simulink model "control_pos_6dof_sinMI"  (R2023b)
settings: Solver=ode45  StartTime=0.0  StopTime=tsim  FixedStep=tstep  MaxStep=tstep  RelTol=tstep/10
undefined symbols (not defined in the file): a0, a1, robot_params, t_qeq_init, t_tr_init, tau_L, tr_ref
(part 2 of 7)

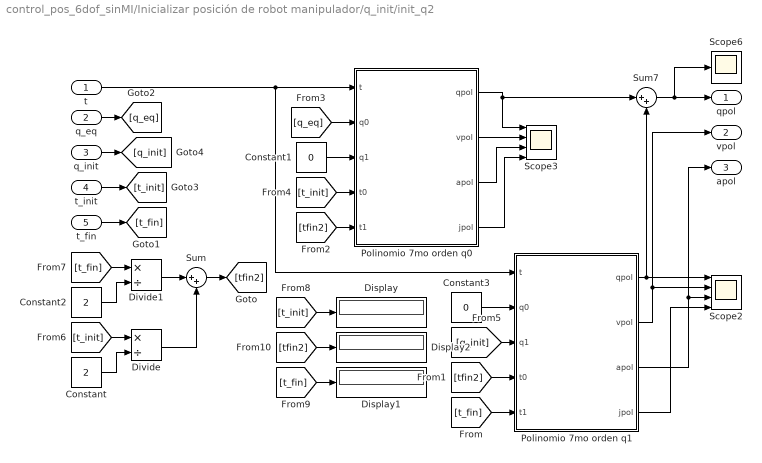
== system control_pos_6dof_sinMI/Inicializar posición de robot manipulador/q_init/init_q2 ==
  t : Inport
  q_eq : Inport  Port=2
  q_init : Inport  Port=3
  t_init : Inport  Port=4
  t_fin : Inport  Port=5
  Constant : Constant  Value=2
  Constant1 : Constant  Value=0
  Constant2 : Constant  Value=2
  Constant3 : Constant  Value=0
  Display : Display
  Display1 : Display
  Display2 : Display
  Divide : Product  Inputs=*/
  Divide1 : Product  Inputs=*/
  Polinomio 7mo orden q0 : MATLAB Function  TreatAsAtomicUnit=on
  Polinomio 7mo orden q1 : MATLAB Function  TreatAsAtomicUnit=on
  Scope2 : Scope  NumInputPorts=4
  Scope3 : Scope  NumInputPorts=4
  Scope6 : Scope
  Sum : Sum  Inputs=|++
  Sum7 : Sum  Inputs=|++
  qpol : Outport
  vpol : Outport  Port=2
  apol : Outport  Port=3
  wires:
  [tfin2] -> Polinomio 7mo orden q0/5(t1)
  t/1 -> Polinomio 7mo orden q1/1(t), Polinomio 7mo orden q0/1(t)
  t_fin/1 -> [t_fin]
  Polinomio 7mo orden q0/1(qpol) -> Sum7/1, Scope3/1
  Polinomio 7mo orden q1/1(qpol) -> Scope2/1, Sum7/2
  [tfin2] -> Polinomio 7mo orden q1/4(t0)
  [t_fin] -> Polinomio 7mo orden q1/5(t1)
  q_eq/1 -> [q_eq]
  q_init/1 -> [q_init]
  [q_eq] -> Polinomio 7mo orden q0/2(q0)
  [q_init] -> Polinomio 7mo orden q1/3(q1)
  Constant1/1 -> Polinomio 7mo orden q0/3(q1)
  Constant3/1 -> Polinomio 7mo orden q1/2(q0)
  Sum7/1 -> qpol/1, Scope6/1
  t_init/1 -> [t_init]
  [t_init] -> Polinomio 7mo orden q0/4(t0)
  Sum/1 -> [tfin2]
  [t_init] -> Display/1
  [t_fin] -> Display1/1
  [tfin2] -> Display2/1
  Divide/1 -> Sum/2
  Constant/1 -> Divide/2
  Divide1/1 -> Sum/1
  Constant2/1 -> Divide1/2
  [t_fin] -> Divide1/1
  [t_init] -> Divide/1
  Polinomio 7mo orden q1/2(vpol) -> vpol/1, Scope2/2
  Polinomio 7mo orden q1/3(apol) -> apol/1, Scope2/3
  Polinomio 7mo orden q1/4(jpol) -> Scope2/4
  Polinomio 7mo orden q0/2(vpol) -> Scope3/2
  Polinomio 7mo orden q0/3(apol) -> Scope3/3
  Polinomio 7mo orden q0/4(jpol) -> Scope3/4

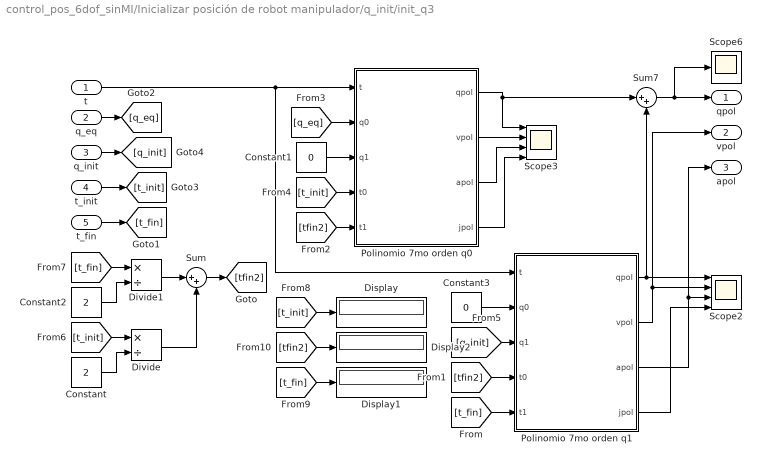
== system control_pos_6dof_sinMI/Inicializar posición de robot manipulador/q_init/init_q3 ==
  t : Inport
  q_eq : Inport  Port=2
  q_init : Inport  Port=3
  t_init : Inport  Port=4
  t_fin : Inport  Port=5
  Constant : Constant  Value=2
  Constant1 : Constant  Value=0
  Constant2 : Constant  Value=2
  Constant3 : Constant  Value=0
  Display : Display
  Display1 : Display
  Display2 : Display
  Divide : Product  Inputs=*/
  Divide1 : Product  Inputs=*/
  Polinomio 7mo orden q0 : MATLAB Function  TreatAsAtomicUnit=on
  Polinomio 7mo orden q1 : MATLAB Function  TreatAsAtomicUnit=on
  Scope2 : Scope  NumInputPorts=4
  Scope3 : Scope  NumInputPorts=4
  Scope6 : Scope
  Sum : Sum  Inputs=|++
  Sum7 : Sum  Inputs=|++
  qpol : Outport
  vpol : Outport  Port=2
  apol : Outport  Port=3
  wires:
  [tfin2] -> Polinomio 7mo orden q0/5(t1)
  t/1 -> Polinomio 7mo orden q1/1(t), Polinomio 7mo orden q0/1(t)
  t_fin/1 -> [t_fin]
  Polinomio 7mo orden q0/1(qpol) -> Sum7/1, Scope3/1
  Polinomio 7mo orden q1/1(qpol) -> Scope2/1, Sum7/2
  [tfin2] -> Polinomio 7mo orden q1/4(t0)
  [t_fin] -> Polinomio 7mo orden q1/5(t1)
  q_eq/1 -> [q_eq]
  q_init/1 -> [q_init]
  [q_eq] -> Polinomio 7mo orden q0/2(q0)
  [q_init] -> Polinomio 7mo orden q1/3(q1)
  Constant1/1 -> Polinomio 7mo orden q0/3(q1)
  Constant3/1 -> Polinomio 7mo orden q1/2(q0)
  Sum7/1 -> qpol/1, Scope6/1
  t_init/1 -> [t_init]
  [t_init] -> Polinomio 7mo orden q0/4(t0)
  Sum/1 -> [tfin2]
  [t_init] -> Display/1
  [t_fin] -> Display1/1
  [tfin2] -> Display2/1
  Divide/1 -> Sum/2
  Constant/1 -> Divide/2
  Divide1/1 -> Sum/1
  Constant2/1 -> Divide1/2
  [t_fin] -> Divide1/1
  [t_init] -> Divide/1
  Polinomio 7mo orden q1/2(vpol) -> vpol/1, Scope2/2
  Polinomio 7mo orden q1/3(apol) -> apol/1, Scope2/3
  Polinomio 7mo orden q1/4(jpol) -> Scope2/4
  Polinomio 7mo orden q0/2(vpol) -> Scope3/2
  Polinomio 7mo orden q0/3(apol) -> Scope3/3
  Polinomio 7mo orden q0/4(jpol) -> Scope3/4

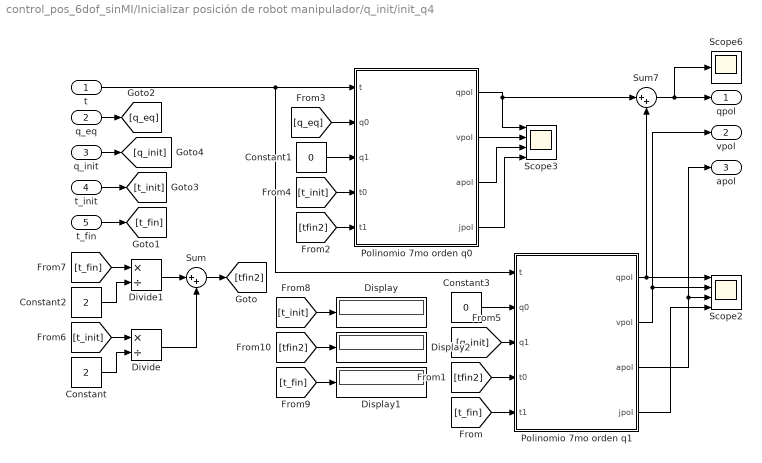
== system control_pos_6dof_sinMI/Inicializar posición de robot manipulador/q_init/init_q4 ==
  t : Inport
  q_eq : Inport  Port=2
  q_init : Inport  Port=3
  t_init : Inport  Port=4
  t_fin : Inport  Port=5
  Constant : Constant  Value=2
  Constant1 : Constant  Value=0
  Constant2 : Constant  Value=2
  Constant3 : Constant  Value=0
  Display : Display
  Display1 : Display
  Display2 : Display
  Divide : Product  Inputs=*/
  Divide1 : Product  Inputs=*/
  Polinomio 7mo orden q0 : MATLAB Function  TreatAsAtomicUnit=on
  Polinomio 7mo orden q1 : MATLAB Function  TreatAsAtomicUnit=on
  Scope2 : Scope  NumInputPorts=4
  Scope3 : Scope  NumInputPorts=4
  Scope6 : Scope
  Sum : Sum  Inputs=|++
  Sum7 : Sum  Inputs=|++
  qpol : Outport
  vpol : Outport  Port=2
  apol : Outport  Port=3
  wires:
  [tfin2] -> Polinomio 7mo orden q0/5(t1)
  t/1 -> Polinomio 7mo orden q1/1(t), Polinomio 7mo orden q0/1(t)
  t_fin/1 -> [t_fin]
  Polinomio 7mo orden q0/1(qpol) -> Sum7/1, Scope3/1
  Polinomio 7mo orden q1/1(qpol) -> Scope2/1, Sum7/2
  [tfin2] -> Polinomio 7mo orden q1/4(t0)
  [t_fin] -> Polinomio 7mo orden q1/5(t1)
  q_eq/1 -> [q_eq]
  q_init/1 -> [q_init]
  [q_eq] -> Polinomio 7mo orden q0/2(q0)
  [q_init] -> Polinomio 7mo orden q1/3(q1)
  Constant1/1 -> Polinomio 7mo orden q0/3(q1)
  Constant3/1 -> Polinomio 7mo orden q1/2(q0)
  Sum7/1 -> qpol/1, Scope6/1
  t_init/1 -> [t_init]
  [t_init] -> Polinomio 7mo orden q0/4(t0)
  Sum/1 -> [tfin2]
  [t_init] -> Display/1
  [t_fin] -> Display1/1
  [tfin2] -> Display2/1
  Divide/1 -> Sum/2
  Constant/1 -> Divide/2
  Divide1/1 -> Sum/1
  Constant2/1 -> Divide1/2
  [t_fin] -> Divide1/1
  [t_init] -> Divide/1
  Polinomio 7mo orden q1/2(vpol) -> vpol/1, Scope2/2
  Polinomio 7mo orden q1/3(apol) -> apol/1, Scope2/3
  Polinomio 7mo orden q1/4(jpol) -> Scope2/4
  Polinomio 7mo orden q0/2(vpol) -> Scope3/2
  Polinomio 7mo orden q0/3(apol) -> Scope3/3
  Polinomio 7mo orden q0/4(jpol) -> Scope3/4

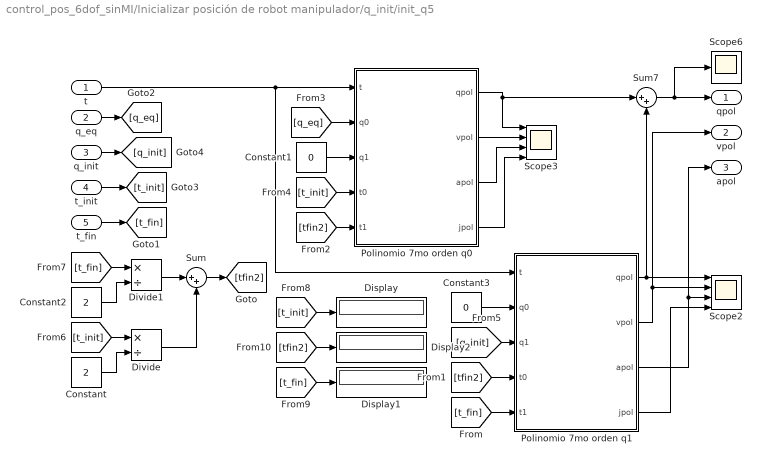
== system control_pos_6dof_sinMI/Inicializar posición de robot manipulador/q_init/init_q5 ==
  t : Inport
  q_eq : Inport  Port=2
  q_init : Inport  Port=3
  t_init : Inport  Port=4
  t_fin : Inport  Port=5
  Constant : Constant  Value=2
  Constant1 : Constant  Value=0
  Constant2 : Constant  Value=2
  Constant3 : Constant  Value=0
  Display : Display
  Display1 : Display
  Display2 : Display
  Divide : Product  Inputs=*/
  Divide1 : Product  Inputs=*/
  Polinomio 7mo orden q0 : MATLAB Function  TreatAsAtomicUnit=on
  Polinomio 7mo orden q1 : MATLAB Function  TreatAsAtomicUnit=on
  Scope2 : Scope  NumInputPorts=4
  Scope3 : Scope  NumInputPorts=4
  Scope6 : Scope
  Sum : Sum  Inputs=|++
  Sum7 : Sum  Inputs=|++
  qpol : Outport
  vpol : Outport  Port=2
  apol : Outport  Port=3
  wires:
  [tfin2] -> Polinomio 7mo orden q0/5(t1)
  t/1 -> Polinomio 7mo orden q1/1(t), Polinomio 7mo orden q0/1(t)
  t_fin/1 -> [t_fin]
  Polinomio 7mo orden q0/1(qpol) -> Sum7/1, Scope3/1
  Polinomio 7mo orden q1/1(qpol) -> Scope2/1, Sum7/2
  [tfin2] -> Polinomio 7mo orden q1/4(t0)
  [t_fin] -> Polinomio 7mo orden q1/5(t1)
  q_eq/1 -> [q_eq]
  q_init/1 -> [q_init]
  [q_eq] -> Polinomio 7mo orden q0/2(q0)
  [q_init] -> Polinomio 7mo orden q1/3(q1)
  Constant1/1 -> Polinomio 7mo orden q0/3(q1)
  Constant3/1 -> Polinomio 7mo orden q1/2(q0)
  Sum7/1 -> qpol/1, Scope6/1
  t_init/1 -> [t_init]
  [t_init] -> Polinomio 7mo orden q0/4(t0)
  Sum/1 -> [tfin2]
  [t_init] -> Display/1
  [t_fin] -> Display1/1
  [tfin2] -> Display2/1
  Divide/1 -> Sum/2
  Constant/1 -> Divide/2
  Divide1/1 -> Sum/1
  Constant2/1 -> Divide1/2
  [t_fin] -> Divide1/1
  [t_init] -> Divide/1
  Polinomio 7mo orden q1/2(vpol) -> vpol/1, Scope2/2
  Polinomio 7mo orden q1/3(apol) -> apol/1, Scope2/3
  Polinomio 7mo orden q1/4(jpol) -> Scope2/4
  Polinomio 7mo orden q0/2(vpol) -> Scope3/2
  Polinomio 7mo orden q0/3(apol) -> Scope3/3
  Polinomio 7mo orden q0/4(jpol) -> Scope3/4

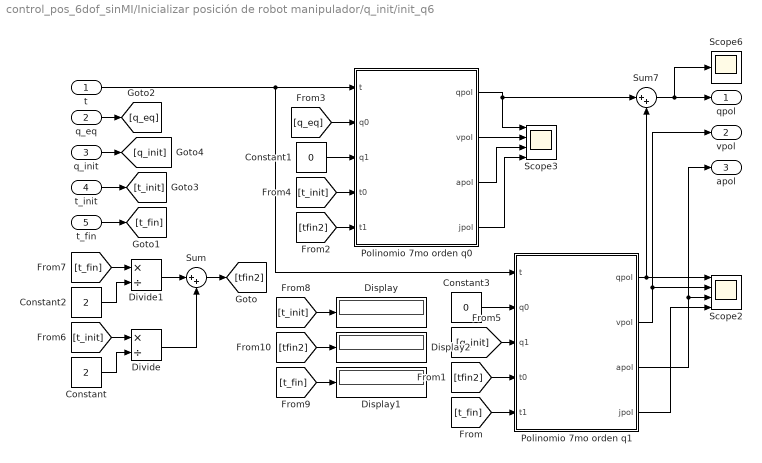
== system control_pos_6dof_sinMI/Inicializar posición de robot manipulador/q_init/init_q6 ==
  t : Inport
  q_eq : Inport  Port=2
  q_init : Inport  Port=3
  t_init : Inport  Port=4
  t_fin : Inport  Port=5
  Constant : Constant  Value=2
  Constant1 : Constant  Value=0
  Constant2 : Constant  Value=2
  Constant3 : Constant  Value=0
  Display : Display
  Display1 : Display
  Display2 : Display
  Divide : Product  Inputs=*/
  Divide1 : Product  Inputs=*/
  Polinomio 7mo orden q0 : MATLAB Function  TreatAsAtomicUnit=on
  Polinomio 7mo orden q1 : MATLAB Function  TreatAsAtomicUnit=on
  Scope2 : Scope  NumInputPorts=4
  Scope3 : Scope  NumInputPorts=4
  Scope6 : Scope
  Sum : Sum  Inputs=|++
  Sum7 : Sum  Inputs=|++
  qpol : Outport
  vpol : Outport  Port=2
  apol : Outport  Port=3
  wires:
  [tfin2] -> Polinomio 7mo orden q0/5(t1)
  t/1 -> Polinomio 7mo orden q1/1(t), Polinomio 7mo orden q0/1(t)
  t_fin/1 -> [t_fin]
  Polinomio 7mo orden q0/1(qpol) -> Sum7/1, Scope3/1
  Polinomio 7mo orden q1/1(qpol) -> Scope2/1, Sum7/2
  [tfin2] -> Polinomio 7mo orden q1/4(t0)
  [t_fin] -> Polinomio 7mo orden q1/5(t1)
  q_eq/1 -> [q_eq]
  q_init/1 -> [q_init]
  [q_eq] -> Polinomio 7mo orden q0/2(q0)
  [q_init] -> Polinomio 7mo orden q1/3(q1)
  Constant1/1 -> Polinomio 7mo orden q0/3(q1)
  Constant3/1 -> Polinomio 7mo orden q1/2(q0)
  Sum7/1 -> qpol/1, Scope6/1
  t_init/1 -> [t_init]
  [t_init] -> Polinomio 7mo orden q0/4(t0)
  Sum/1 -> [tfin2]
  [t_init] -> Display/1
  [t_fin] -> Display1/1
  [tfin2] -> Display2/1
  Divide/1 -> Sum/2
  Constant/1 -> Divide/2
  Divide1/1 -> Sum/1
  Constant2/1 -> Divide1/2
  [t_fin] -> Divide1/1
  [t_init] -> Divide/1
  Polinomio 7mo orden q1/2(vpol) -> vpol/1, Scope2/2
  Polinomio 7mo orden q1/3(apol) -> apol/1, Scope2/3
  Polinomio 7mo orden q1/4(jpol) -> Scope2/4
  Polinomio 7mo orden q0/2(vpol) -> Scope3/2
  Polinomio 7mo orden q0/3(apol) -> Scope3/3
  Polinomio 7mo orden q0/4(jpol) -> Scope3/4

== system control_pos_6dof_sinMI/Inicializar posición de robot manipulador/q_init_tr/q1 ==
  q_init : Inport
  q_fin : Inport  Port=2
  t_fin : Inport  Port=3
  Clock1 : Clock
  Constant : Constant  Value=pi/4
  Polinomio 7mo orden dq : MATLAB Function  TreatAsAtomicUnit=on
  Sum : Sum  Inputs=|++
  qpol : Outport
  vpol : Outport  Port=2
  apol : Outport  Port=3
  wires:
  Clock1/1 -> Polinomio 7mo orden dq/1(t)
  q_fin/1 -> Polinomio 7mo orden dq/3(q1)
  t_fin/1 -> Sum/1, Polinomio 7mo orden dq/4(t0)
  Polinomio 7mo orden dq/1(qpol) -> qpol/1
  Constant/1 -> Sum/2
  Sum/1 -> Polinomio 7mo orden dq/5(t1)
  q_init/1 -> Polinomio 7mo orden dq/2(q0)
  Polinomio 7mo orden dq/2(vpol) -> vpol/1
  Polinomio 7mo orden dq/3(apol) -> apol/1

== system control_pos_6dof_sinMI/Inicializar posición de robot manipulador/q_init_tr/q2 ==
  q_init : Inport
  q_fin : Inport  Port=2
  t_fin : Inport  Port=3
  Clock1 : Clock
  Constant : Constant  Value=pi/4
  Polinomio 7mo orden dq : MATLAB Function  TreatAsAtomicUnit=on
  Sum : Sum  Inputs=|++
  qpol : Outport
  vpol : Outport  Port=2
  apol : Outport  Port=3
  wires:
  Clock1/1 -> Polinomio 7mo orden dq/1(t)
  q_fin/1 -> Polinomio 7mo orden dq/3(q1)
  t_fin/1 -> Sum/1, Polinomio 7mo orden dq/4(t0)
  Polinomio 7mo orden dq/1(qpol) -> qpol/1
  Constant/1 -> Sum/2
  Sum/1 -> Polinomio 7mo orden dq/5(t1)
  q_init/1 -> Polinomio 7mo orden dq/2(q0)
  Polinomio 7mo orden dq/2(vpol) -> vpol/1
  Polinomio 7mo orden dq/3(apol) -> apol/1

== system control_pos_6dof_sinMI/Inicializar posición de robot manipulador/q_init_tr/q3 ==
  q_init : Inport
  q_fin : Inport  Port=2
  t_fin : Inport  Port=3
  Clock1 : Clock
  Constant : Constant  Value=pi/4
  Polinomio 7mo orden dq : MATLAB Function  TreatAsAtomicUnit=on
  Sum : Sum  Inputs=|++
  qpol : Outport
  vpol : Outport  Port=2
  apol : Outport  Port=3
  wires:
  Clock1/1 -> Polinomio 7mo orden dq/1(t)
  q_fin/1 -> Polinomio 7mo orden dq/3(q1)
  t_fin/1 -> Sum/1, Polinomio 7mo orden dq/4(t0)
  Polinomio 7mo orden dq/1(qpol) -> qpol/1
  Constant/1 -> Sum/2
  Sum/1 -> Polinomio 7mo orden dq/5(t1)
  q_init/1 -> Polinomio 7mo orden dq/2(q0)
  Polinomio 7mo orden dq/2(vpol) -> vpol/1
  Polinomio 7mo orden dq/3(apol) -> apol/1

== system control_pos_6dof_sinMI/Inicializar posición de robot manipulador/q_init_tr/q4 ==
  q_init : Inport
  q_fin : Inport  Port=2
  t_fin : Inport  Port=3
  Clock1 : Clock
  Constant : Constant  Value=pi/4
  Polinomio 7mo orden dq : MATLAB Function  TreatAsAtomicUnit=on
  Sum : Sum  Inputs=|++
  qpol : Outport
  vpol : Outport  Port=2
  apol : Outport  Port=3
  wires:
  Clock1/1 -> Polinomio 7mo orden dq/1(t)
  q_fin/1 -> Polinomio 7mo orden dq/3(q1)
  t_fin/1 -> Sum/1, Polinomio 7mo orden dq/4(t0)
  Polinomio 7mo orden dq/1(qpol) -> qpol/1
  Constant/1 -> Sum/2
  Sum/1 -> Polinomio 7mo orden dq/5(t1)
  q_init/1 -> Polinomio 7mo orden dq/2(q0)
  Polinomio 7mo orden dq/2(vpol) -> vpol/1
  Polinomio 7mo orden dq/3(apol) -> apol/1

== system control_pos_6dof_sinMI/Inicializar posición de robot manipulador/q_init_tr/q5 ==
  q_init : Inport
  q_fin : Inport  Port=2
  t_fin : Inport  Port=3
  Clock1 : Clock
  Constant : Constant  Value=pi/4
  Polinomio 7mo orden dq : MATLAB Function  TreatAsAtomicUnit=on
  Sum : Sum  Inputs=|++
  qpol : Outport
  vpol : Outport  Port=2
  apol : Outport  Port=3
  wires:
  Clock1/1 -> Polinomio 7mo orden dq/1(t)
  q_fin/1 -> Polinomio 7mo orden dq/3(q1)
  t_fin/1 -> Sum/1, Polinomio 7mo orden dq/4(t0)
  Polinomio 7mo orden dq/1(qpol) -> qpol/1
  Constant/1 -> Sum/2
  Sum/1 -> Polinomio 7mo orden dq/5(t1)
  q_init/1 -> Polinomio 7mo orden dq/2(q0)
  Polinomio 7mo orden dq/2(vpol) -> vpol/1
  Polinomio 7mo orden dq/3(apol) -> apol/1

== system control_pos_6dof_sinMI/Inicializar posición de robot manipulador/q_init_tr/q6 ==
  q_init : Inport
  q_fin : Inport  Port=2
  t_fin : Inport  Port=3
  Clock1 : Clock
  Constant : Constant  Value=pi/4
  Polinomio 7mo orden dq : MATLAB Function  TreatAsAtomicUnit=on
  Sum : Sum  Inputs=|++
  qpol : Outport
  vpol : Outport  Port=2
  apol : Outport  Port=3
  wires:
  Clock1/1 -> Polinomio 7mo orden dq/1(t)
  q_fin/1 -> Polinomio 7mo orden dq/3(q1)
  t_fin/1 -> Sum/1, Polinomio 7mo orden dq/4(t0)
  Polinomio 7mo orden dq/1(qpol) -> qpol/1
  Constant/1 -> Sum/2
  Sum/1 -> Polinomio 7mo orden dq/5(t1)
  q_init/1 -> Polinomio 7mo orden dq/2(q0)
  Polinomio 7mo orden dq/2(vpol) -> vpol/1
  Polinomio 7mo orden dq/3(apol) -> apol/1

== matlab function control_pos_6dof_sinMI/xyz to q (referencia)/dr to dq ==
  data: JP input size=[3,6]; dq output size=[6,1]; dr input size=[3,1]
function dq = fcn(JP,dr)

% Pseudoinversa derecha JPinv = zeros(6,3)
JPinv = JP.'*(JP*JP.')^-1;

% Velocidades articulares
dq = JPinv*dr;

== matlab function control_pos_6dof_sinMI/xyz to q (referencia)/Jacobiano ==
  data: robot_params input; q input; JP output
function JP = JP(robot_params,q)

%l1 = robot_params.l(1);
l2 = robot_params.l(2);
l3 = robot_params.l(3);
%l4 = robot_params.l(4);
%l5 = robot_params.l(5);
%l6 = robot_params.l(6);

lc1 = robot_params.lc(1);
lc2 = robot_params.lc(2);
lc3 = robot_params.lc(3);
%lc4 = robot_params.lc(4);
%lc5 = robot_params.lc(5);
%lc6 = robot_params.lc(6);

d1 = robot_params.d(1);
%d2 = robot_params.d(2);
%d3 = robot_params.d(3);
d4 = robot_params.d(4);
d5 = robot_params.d(5);
%d6 = robot_params.d(6);

dc1 = robot_params.dc(1);
%dc2 = robot_params.dc(2);
%dc3 = robot_params.dc(3);
dc4 = robot_params.dc(4);
dc5 = robot_params.dc(5);
dc6 = robot_params.dc(6);

q1 = q(1);
q2 = q(2);
q3 = q(3);
q4 = q(4);
q5 = q(5);
%q6 = q(6);

% Cinematica diferencial %%%%%%%%%%%%%%%%%%%%%%%%%%%%%%%%%%%%%%%%%%%%%%%%%%

JP = zeros(3,6);

JP(1,1) = -cos(q1)*(d1 + l3*sin(q2 + q3) + l2*sin(q2) - d5*cos(q2 + q3 + q4) - dc6*sin(q2 + q3 + q4)*sin(q5));
JP(1,2) = -cos(q1)*(d1 - dc1 + l3*sin(q2 + q3) + l2*sin(q2) - d5*cos(q2 + q3 + q4) - dc6*sin(q2 + q3 + q4)*sin(q5));
JP(1,3) = cos(q1)*(lc2*sin(q2) - l2*sin(q2) - l3*sin(q2 + q3) + d5*cos(q2 + q3 + q4) + dc6*sin(q2 + q3 + q4)*sin(q5));
JP(1,4) = - cos(q2 + q3 + q4)*(dc6*(cos(q1)*cos(q5) + cos(q2 + q3 + q4)*sin(q1)*sin(q5)) + d4*cos(q1) - sin(q1)*(l3*cos(q2 + q3) + l2*cos(q2)) + sin(q1)*(lc3*cos(q2 + q3) + l2*cos(q2)) - d5*sin(q2 + q3 + q4)*sin(q1)) - sin(q2 + q3 + q4)*sin(q1)*(lc3*sin(q2 + q3) - l3*sin(q2 + q3) + d5*cos(q2 + q3 + q4) + dc6*sin(q2 + q3 + q4)*sin(q5));
JP(1,5) = d5*sin(q1)*sin(q5) + d5*cos(q2 + q3 + q4)*cos(q1)*cos(q5) - d4*sin(q2 + q3 + q4)*cos(q1)*sin(q5) + dc4*sin(q2 + q3 + q4)*cos(q1)*sin(q5);
JP(1,6) = (d5 - dc5)*(sin(q1)*sin(q5) + cos(q2 + q3 + q4)*cos(q1)*cos(q5));

JP(2,1) = -sin(q1)*(d1 + l3*sin(q2 + q3) + l2*sin(q2) - d5*cos(q2 + q3 + q4) - dc6*sin(q2 + q3 + q4)*sin(q5));
JP(2,2) = -sin(q1)*(d1 - dc1 + l3*sin(q2 + q3) + l2*sin(q2) - d5*cos(q2 + q3 + q4) - dc6*sin(q2 + q3 + q4)*sin(q5));
JP(2,3) = sin(q1)*(lc2*sin(q2) - l2*sin(q2) - l3*sin(q2 + q3) + d5*cos(q2 + q3 + q4) + dc6*sin(q2 + q3 + q4)*sin(q5));
JP(2,4) = sin(q2 + q3 + q4)*cos(q1)*(lc3*sin(q2 + q3) - l3*sin(q2 + q3) + d5*cos(q2 + q3 + q4) + dc6*sin(q2 + q3 + q4)*sin(q5)) - cos(q2 + q3 + q4)*(dc6*(cos(q5)*sin(q1) - cos(q2 + q3 + q4)*cos(q1)*sin(q5)) + cos(q1)*(l3*cos(q2 + q3) + l2*cos(q2)) - cos(q1)*(lc3*cos(q2 + q3) + l2*cos(q2)) + d4*sin(q1) + d5*sin(q2 + q3 + q4)*cos(q1));
JP(2,5) = d5*cos(q2 + q3 + q4)*cos(q5)*sin(q1) - d5*cos(q1)*sin(q5) - d4*sin(q2 + q3 + q4)*sin(q1)*sin(q5) + dc4*sin(q2 + q3 + q4)*sin(q1)*sin(q5);
JP(2,6) = -(d5 - dc5)*(cos(q1)*sin(q5) - cos(q2 + q3 + q4)*cos(q5)*sin(q1));

JP(3,1) = l3*cos(q2 + q3) - (dc6*sin(q2 + q3 + q4 + q5))/2 + l2*cos(q2) + (dc6*sin(q2 + q3 + q4 - q5))/2 + d5*sin(q2 + q3 + q4);
JP(3,2) = l3*cos(q2 + q3) - (dc6*sin(q2 + q3 + q4 + q5))/2 - lc1 + l2*cos(q2) + (dc6*sin(q2 + q3 + q4 - q5))/2 + d5*sin(q2 + q3 + q4);
JP(3,3) = l3*cos(q2 + q3) - (dc6*sin(q2 + q3 + q4 + q5))/2 + l2*cos(q2) - lc2*cos(q2) + (dc6*sin(q2 + q3 + q4 - q5))/2 + d5*sin(q2 + q3 + q4);
JP(3,4) = - (dc6*sin(q2 + q3 + q4 + q5))/2 - (dc6*sin(q2 + q3 + q4 - q5))/2 - d4*sin(q2 + q3 + q4);
JP(3,5) = d4*cos(q2 + q3 + q4)*sin(q5) + d5*sin(q2 + q3 + q4)*cos(q5) - dc4*cos(q2 + q3 + q4)*sin(q5);
JP(3,6) = sin(q2 + q3 + q4)*cos(q5)*(d5 - dc5);

== matlab function control_pos_6dof_sinMI/xyz to q (referencia)/derivada Jacobiano ==
  data: robot_params input; q input; dJP output; dq input
function dJP = dJP(robot_params,q,dq)

%l1 = robot_params.l(1);
l2 = robot_params.l(2);
l3 = robot_params.l(3);
%l4 = robot_params.l(4);
%l5 = robot_params.l(5);
%l6 = robot_params.l(6);

lc1 = robot_params.lc(1);
lc2 = robot_params.lc(2);
lc3 = robot_params.lc(3);
%lc4 = robot_params.lc(4);
%lc5 = robot_params.lc(5);
%lc6 = robot_params.lc(6);

d1 = robot_params.d(1);
%d2 = robot_params.d(2);
%d3 = robot_params.d(3);
d4 = robot_params.d(4);
d5 = robot_params.d(5);
%d6 = robot_params.d(6);

dc1 = robot_params.dc(1);
%dc2 = robot_params.dc(2);
%dc3 = robot_params.dc(3);
dc4 = robot_params.dc(4);
dc5 = robot_params.dc(5);
dc6 = robot_params.dc(6);

dq1 = dq(1);
dq2 = dq(2);
dq3 = dq(3);
dq4 = dq(4);
dq5 = dq(5);
%dq6 = dq(6);

q1 = q(1);
q2 = q(2);
q3 = q(3);
q4 = q(4);
q5 = q(5);
%q6 = q(6);

dJP = zeros(3,6);

dJP(1,1) = dq1*sin(q1)*(d1 + l3*sin(q2 + q3) + l2*sin(q2) - d5*cos(q2 + q3 + q4) - dc6*sin(q2 + q3 + q4)*sin(q5)) - dq3*cos(q1)*(l3*cos(q2 + q3) + d5*sin(q2 + q3 + q4) - dc6*cos(q2 + q3 + q4)*sin(q5)) - dq4*cos(q1)*(d5*sin(q2 + q3 + q4) - dc6*cos(q2 + q3 + q4)*sin(q5)) - dq2*cos(q1)*(l3*cos(q2 + q3) + l2*cos(q2) + d5*sin(q2 + q3 + q4) - dc6*cos(q2 + q3 + q4)*sin(q5)) + dc6*dq5*sin(q2 + q3 + q4)*cos(q1)*cos(q5);
dJP(1,2) = dq1*sin(q1)*(d1 - dc1 + l3*sin(q2 + q3) + l2*sin(q2) - d5*cos(q2 + q3 + q4) - dc6*sin(q2 + q3 + q4)*sin(q5)) - dq3*cos(q1)*(l3*cos(q2 + q3) + d5*sin(q2 + q3 + q4) - dc6*cos(q2 + q3 + q4)*sin(q5)) - dq4*cos(q1)*(d5*sin(q2 + q3 + q4) - dc6*cos(q2 + q3 + q4)*sin(q5)) - dq2*cos(q1)*(l3*cos(q2 + q3) + l2*cos(q2) + d5*sin(q2 + q3 + q4) - dc6*cos(q2 + q3 + q4)*sin(q5)) + dc6*dq5*sin(q2 + q3 + q4)*cos(q1)*cos(q5);
dJP(1,3) = dc6*dq5*sin(q2 + q3 + q4)*cos(q1)*cos(q5) - dq2*cos(q1)*(l3*cos(q2 + q3) + l2*cos(q2) - lc2*cos(q2) + d5*sin(q2 + q3 + q4) - dc6*cos(q2 + q3 + q4)*sin(q5)) - dq1*sin(q1)*(lc2*sin(q2) - l2*sin(q2) - l3*sin(q2 + q3) + d5*cos(q2 + q3 + q4) + dc6*sin(q2 + q3 + q4)*sin(q5)) - dq4*cos(q1)*(d5*sin(q2 + q3 + q4) - dc6*cos(q2 + q3 + q4)*sin(q5)) - dq3*cos(q1)*(l3*cos(q2 + q3) + d5*sin(q2 + q3 + q4) - dc6*cos(q2 + q3 + q4)*sin(q5));
dJP(1,4) = dq1*l3*cos(q1)*cos(q4) - dq1*lc3*cos(q1)*cos(q4) - dc6*dq1*cos(q1)*sin(q5) - dc6*dq5*cos(q5)*sin(q1) - dq4*l3*sin(q1)*sin(q4) + dq4*lc3*sin(q1)*sin(q4) + d4*dq1*cos(q2)*cos(q3)*cos(q4)*sin(q1) + d4*dq2*cos(q1)*cos(q2)*cos(q3)*sin(q4) + d4*dq2*cos(q1)*cos(q2)*cos(q4)*sin(q3) + d4*dq2*cos(q1)*cos(q3)*cos(q4)*sin(q2) + d4*dq3*cos(q1)*cos(q2)*cos(q3)*sin(q4) + d4*dq3*cos(q1)*cos(q2)*cos(q4)*sin(q3) + d4*dq3*cos(q1)*cos(q3)*cos(q4)*sin(q2) + d4*dq4*cos(q1)*cos(q2)*cos(q3)*sin(q4) + d4*dq4*cos(q1)*cos(q2)*cos(q4)*sin(q3) + d4*dq4*cos(q1)*cos(q3)*cos(q4)*sin(q2) - d4*dq1*cos(q2)*sin(q1)*sin(q3)*sin(q4) - d4*dq1*cos(q3)*sin(q1)*sin(q2)*sin(q4) - d4*dq1*cos(q4)*sin(q1)*sin(q2)*sin(q3) - d4*dq2*cos(q1)*sin(q2)*sin(q3)*sin(q4) - d4*dq3*cos(q1)*sin(q2)*sin(q3)*sin(q4) - d4*dq4*cos(q1)*sin(q2)*sin(q3)*sin(q4) + dc6*dq1*cos(q2)*cos(q3)*cos(q4)*cos(q5)*sin(q1) + dc6*dq2*cos(q1)*cos(q2)*cos(q3)*cos(q5)*sin(q4) + dc6*dq2*cos(q1)*cos(q2)*cos(q4)*cos(q5)*sin(q3) + dc6*dq2*cos(q1)*cos(q3)*cos(q4)*cos(q5)*sin(q2) + dc6*dq3*cos(q1)*cos(q2)*cos(q3)*cos(q5)*sin(q4) + dc6*dq3*cos(q1)*cos(q2)*cos(q4)*cos(q5)*sin(q3) + dc6*dq3*cos(q1)*cos(q3)*cos(q4)*cos(q5)*sin(q2) + dc6*dq4*cos(q1)*cos(q2)*cos(q3)*cos(q5)*sin(q4) + dc6*dq4*cos(q1)*cos(q2)*cos(q4)*cos(q5)*sin(q3) + dc6*dq4*cos(q1)*cos(q3)*cos(q4)*cos(q5)*sin(q2) + dc6*dq5*cos(q1)*cos(q2)*cos(q3)*cos(q4)*sin(q5) - dc6*dq1*cos(q2)*cos(q5)*sin(q1)*sin(q3)*sin(q4) - dc6*dq1*cos(q3)*cos(q5)*sin(q1)*sin(q2)*sin(q4) - dc6*dq1*cos(q4)*cos(q5)*sin(q1)*sin(q2)*sin(q3) - dc6*dq2*cos(q1)*cos(q5)*sin(q2)*sin(q3)*sin(q4) - dc6*dq3*cos(q1)*cos(q5)*sin(q2)*sin(q3)*sin(q4) - dc6*dq4*cos(q1)*cos(q5)*sin(q2)*sin(q3)*sin(q4) - dc6*dq5*cos(q1)*cos(q2)*sin(q3)*sin(q4)*sin(q5) - dc6*dq5*cos(q1)*cos(q3)*sin(q2)*sin(q4)*sin(q5) - dc6*dq5*cos(q1)*cos(q4)*sin(q2)*sin(q3)*sin(q5);
dJP(1,5) = dq5*(d5*cos(q5)*sin(q1) - d4*sin(q2 + q3 + q4)*cos(q1)*cos(q5) - d5*cos(q2 + q3 + q4)*cos(q1)*sin(q5) + dc4*sin(q2 + q3 + q4)*cos(q1)*cos(q5)) + dq1*(d5*cos(q1)*sin(q5) - d5*cos(q2 + q3 + q4)*cos(q5)*sin(q1) + d4*sin(q2 + q3 + q4)*sin(q1)*sin(q5) - dc4*sin(q2 + q3 + q4)*sin(q1)*sin(q5)) - dq2*cos(q1)*(d4*cos(q2 + q3 + q4)*sin(q5) + d5*sin(q2 + q3 + q4)*cos(q5) - dc4*cos(q2 + q3 + q4)*sin(q5)) - dq3*cos(q1)*(d4*cos(q2 + q3 + q4)*sin(q5) + d5*sin(q2 + q3 + q4)*cos(q5) - dc4*cos(q2 + q3 + q4)*sin(q5)) - dq4*cos(q1)*(d4*cos(q2 + q3 + q4)*sin(q5) + d5*sin(q2 + q3 + q4)*cos(q5) - dc4*cos(q2 + q3 + q4)*sin(q5));
dJP(1,6) = dq1*(d5 - dc5)*(cos(q1)*sin(q5) - cos(q2 + q3 + q4)*cos(q5)*sin(q1)) + dq5*(d5 - dc5)*(cos(q5)*sin(q1) - cos(q2 + q3 + q4)*cos(q1)*sin(q5)) - dq2*sin(q2 + q3 + q4)*cos(q1)*cos(q5)*(d5 - dc5) - dq3*sin(q2 + q3 + q4)*cos(q1)*cos(q5)*(d5 - dc5) - dq4*sin(q2 + q3 + q4)*cos(q1)*cos(q5)*(d5 - dc5);

dJP(2,1) = dc6*dq5*sin(q2 + q3 + q4)*cos(q5)*sin(q1) - dq1*cos(q1)*(d1 + l3*sin(q2 + q3) + l2*sin(q2) - d5*cos(q2 + q3 + q4) - dc6*sin(q2 + q3 + q4)*sin(q5)) - dq4*sin(q1)*(d5*sin(q2 + q3 + q4) - dc6*cos(q2 + q3 + q4)*sin(q5)) - dq2*sin(q1)*(l3*cos(q2 + q3) + l2*cos(q2) + d5*sin(q2 + q3 + q4) - dc6*cos(q2 + q3 + q4)*sin(q5)) - dq3*sin(q1)*(l3*cos(q2 + q3) + d5*sin(q2 + q3 + q4) - dc6*cos(q2 + q3 + q4)*sin(q5));
dJP(2,2) = dc6*dq5*sin(q2 + q3 + q4)*cos(q5)*sin(q1) - dq4*sin(q1)*(d5*sin(q2 + q3 + q4) - dc6*cos(q2 + q3 + q4)*sin(q5)) - dq2*sin(q1)*(l3*cos(q2 + q3) + l2*cos(q2) + d5*sin(q2 + q3 + q4) - dc6*cos(q2 + q3 + q4)*sin(q5)) - dq1*cos(q1)*(d1 - dc1 + l3*sin(q2 + q3) + l2*sin(q2) - d5*cos(q2 + q3 + q4) - dc6*sin(q2 + q3 + q4)*sin(q5)) - dq3*sin(q1)*(l3*cos(q2 + q3) + d5*sin(q2 + q3 + q4) - dc6*cos(q2 + q3 + q4)*sin(q5));
dJP(2,3) = dq1*cos(q1)*(lc2*sin(q2) - l2*sin(q2) - l3*sin(q2 + q3) + d5*cos(q2 + q3 + q4) + dc6*sin(q2 + q3 + q4)*sin(q5)) - dq2*sin(q1)*(l3*cos(q2 + q3) + l2*cos(q2) - lc2*cos(q2) + d5*sin(q2 + q3 + q4) - dc6*cos(q2 + q3 + q4)*sin(q5)) - dq3*sin(q1)*(l3*cos(q2 + q3) + d5*sin(q2 + q3 + q4) - dc6*cos(q2 + q3 + q4)*sin(q5)) - dq4*sin(q1)*(d5*sin(q2 + q3 + q4) - dc6*cos(q2 + q3 + q4)*sin(q5)) + dc6*dq5*sin(q2 + q3 + q4)*cos(q5)*sin(q1);
dJP(2,4) = dc6*dq5*cos(q1)*cos(q5) + dq1*l3*cos(q4)*sin(q1) + dq4*l3*cos(q1)*sin(q4) - dq1*lc3*cos(q4)*sin(q1) - dq4*lc3*cos(q1)*sin(q4) - dc6*dq1*sin(q1)*sin(q5) - d4*dq1*cos(q1)*cos(q2)*cos(q3)*cos(q4) + d4*dq1*cos(q1)*cos(q2)*sin(q3)*sin(q4) + d4*dq1*cos(q1)*cos(q3)*sin(q2)*sin(q4) + d4*dq1*cos(q1)*cos(q4)*sin(q2)*sin(q3) + d4*dq2*cos(q2)*cos(q3)*sin(q1)*sin(q4) + d4*dq2*cos(q2)*cos(q4)*sin(q1)*sin(q3) + d4*dq2*cos(q3)*cos(q4)*sin(q1)*sin(q2) + d4*dq3*cos(q2)*cos(q3)*sin(q1)*sin(q4) + d4*dq3*cos(q2)*cos(q4)*sin(q1)*sin(q3) + d4*dq3*cos(q3)*cos(q4)*sin(q1)*sin(q2) + d4*dq4*cos(q2)*cos(q3)*sin(q1)*sin(q4) + d4*dq4*cos(q2)*cos(q4)*sin(q1)*sin(q3) + d4*dq4*cos(q3)*cos(q4)*sin(q1)*sin(q2) - d4*dq2*sin(q1)*sin(q2)*sin(q3)*sin(q4) - d4*dq3*sin(q1)*sin(q2)*sin(q3)*sin(q4) - d4*dq4*sin(q1)*sin(q2)*sin(q3)*sin(q4) - dc6*dq1*cos(q1)*cos(q2)*cos(q3)*cos(q4)*cos(q5) + dc6*dq1*cos(q1)*cos(q2)*cos(q5)*sin(q3)*sin(q4) + dc6*dq1*cos(q1)*cos(q3)*cos(q5)*sin(q2)*sin(q4) + dc6*dq1*cos(q1)*cos(q4)*cos(q5)*sin(q2)*sin(q3) + dc6*dq2*cos(q2)*cos(q3)*cos(q5)*sin(q1)*sin(q4) + dc6*dq2*cos(q2)*cos(q4)*cos(q5)*sin(q1)*sin(q3) + dc6*dq2*cos(q3)*cos(q4)*cos(q5)*sin(q1)*sin(q2) + dc6*dq3*cos(q2)*cos(q3)*cos(q5)*sin(q1)*sin(q4) + dc6*dq3*cos(q2)*cos(q4)*cos(q5)*sin(q1)*sin(q3) + dc6*dq3*cos(q3)*cos(q4)*cos(q5)*sin(q1)*sin(q2) + dc6*dq4*cos(q2)*cos(q3)*cos(q5)*sin(q1)*sin(q4) + dc6*dq4*cos(q2)*cos(q4)*cos(q5)*sin(q1)*sin(q3) + dc6*dq4*cos(q3)*cos(q4)*cos(q5)*sin(q1)*sin(q2) + dc6*dq5*cos(q2)*cos(q3)*cos(q4)*sin(q1)*sin(q5) - dc6*dq2*cos(q5)*sin(q1)*sin(q2)*sin(q3)*sin(q4) - dc6*dq3*cos(q5)*sin(q1)*sin(q2)*sin(q3)*sin(q4) - dc6*dq4*cos(q5)*sin(q1)*sin(q2)*sin(q3)*sin(q4) - dc6*dq5*cos(q2)*sin(q1)*sin(q3)*sin(q4)*sin(q5) - dc6*dq5*cos(q3)*sin(q1)*sin(q2)*sin(q4)*sin(q5) - dc6*dq5*cos(q4)*sin(q1)*sin(q2)*sin(q3)*sin(q5);
dJP(2,5) = dq1*(d5*sin(q1)*sin(q5) + d5*cos(q2 + q3 + q4)*cos(q1)*cos(q5) - d4*sin(q2 + q3 + q4)*cos(q1)*sin(q5) + dc4*sin(q2 + q3 + q4)*cos(q1)*sin(q5)) - dq5*(d5*cos(q1)*cos(q5) + d4*sin(q2 + q3 + q4)*cos(q5)*sin(q1) + d5*cos(q2 + q3 + q4)*sin(q1)*sin(q5) - dc4*sin(q2 + q3 + q4)*cos(q5)*sin(q1)) - dq2*sin(q1)*(d4*cos(q2 + q3 + q4)*sin(q5) + d5*sin(q2 + q3 + q4)*cos(q5) - dc4*cos(q2 + q3 + q4)*sin(q5)) - dq3*sin(q1)*(d4*cos(q2 + q3 + q4)*sin(q5) + d5*sin(q2 + q3 + q4)*cos(q5) - dc4*cos(q2 + q3 + q4)*sin(q5)) - dq4*sin(q1)*(d4*cos(q2 + q3 + q4)*sin(q5) + d5*sin(q2 + q3 + q4)*cos(q5) - dc4*cos(q2 + q3 + q4)*sin(q5));
dJP(2,6) = dq1*(d5 - dc5)*(sin(q1)*sin(q5) + cos(q2 + q3 + q4)*cos(q1)*cos(q5)) - dq5*(d5 - dc5)*(cos(q1)*cos(q5) + cos(q2 + q3 + q4)*sin(q1)*sin(q5)) - dq2*sin(q2 + q3 + q4)*cos(q5)*sin(q1)*(d5 - dc5) - dq3*sin(q2 + q3 + q4)*cos(q5)*sin(q1)*(d5 - dc5) - dq4*sin(q2 + q3 + q4)*cos(q5)*sin(q1)*(d5 - dc5);

dJP(3,1) = dq4*((dc6*cos(q2 + q3 + q4 - q5))/2 - (dc6*cos(q2 + q3 + q4 + q5))/2 + d5*cos(q2 + q3 + q4)) - dq3*((dc6*cos(q2 + q3 + q4 + q5))/2 + l3*sin(q2 + q3) - (dc6*cos(q2 + q3 + q4 - q5))/2 - d5*cos(q2 + q3 + q4)) - dq2*((dc6*cos(q2 + q3 + q4 + q5))/2 + l3*sin(q2 + q3) - (dc6*cos(q2 + q3 + q4 - q5))/2 + l2*sin(q2) - d5*cos(q2 + q3 + q4)) - (dc6*dq5*(cos(q2 + q3 + q4 + q5) + cos(q2 + q3 + q4 - q5)))/2;
dJP(3,2) = dq4*((dc6*cos(q2 + q3 + q4 - q5))/2 - (dc6*cos(q2 + q3 + q4 + q5))/2 + d5*cos(q2 + q3 + q4)) - dq3*((dc6*cos(q2 + q3 + q4 + q5))/2 + l3*sin(q2 + q3) - (dc6*cos(q2 + q3 + q4 - q5))/2 - d5*cos(q2 + q3 + q4)) - dq2*((dc6*cos(q2 + q3 + q4 + q5))/2 + l3*sin(q2 + q3) - (dc6*cos(q2 + q3 + q4 - q5))/2 + l2*sin(q2) - d5*cos(q2 + q3 + q4)) - (dc6*dq5*(cos(q2 + q3 + q4 + q5) + cos(q2 + q3 + q4 - q5)))/2;
dJP(3,3) = dq4*((dc6*cos(q2 + q3 + q4 - q5))/2 - (dc6*cos(q2 + q3 + q4 + q5))/2 + d5*cos(q2 + q3 + q4)) - dq3*((dc6*cos(q2 + q3 + q4 + q5))/2 + l3*sin(q2 + q3) - (dc6*cos(q2 + q3 + q4 - q5))/2 - d5*cos(q2 + q3 + q4)) - dq2*((dc6*cos(q2 + q3 + q4 + q5))/2 + l3*sin(q2 + q3) - (dc6*cos(q2 + q3 + q4 - q5))/2 + l2*sin(q2) - lc2*sin(q2) - d5*cos(q2 + q3 + q4)) - dq5*((dc6*cos(q2 + q3 + q4 + q5))/2 + (dc6*cos(q2 + q3 + q4 - q5))/2);
dJP(3,4) = - dq2*((dc6*cos(q2 + q3 + q4 + q5))/2 + (dc6*cos(q2 + q3 + q4 - q5))/2 + d4*cos(q2 + q3 + q4)) - dq3*((dc6*cos(q2 + q3 + q4 + q5))/2 + (dc6*cos(q2 + q3 + q4 - q5))/2 + d4*cos(q2 + q3 + q4)) - dq4*((dc6*cos(q2 + q3 + q4 + q5))/2 + (dc6*cos(q2 + q3 + q4 - q5))/2 + d4*cos(q2 + q3 + q4)) - (dc6*dq5*(cos(q2 + q3 + q4 + q5) - cos(q2 + q3 + q4 - q5)))/2;
dJP(3,5) = dq2*(d5*cos(q2 + q3 + q4)*cos(q5) - d4*sin(q2 + q3 + q4)*sin(q5) + dc4*sin(q2 + q3 + q4)*sin(q5)) - dq5*(dc4*cos(q2 + q3 + q4)*cos(q5) - d4*cos(q2 + q3 + q4)*cos(q5) + d5*sin(q2 + q3 + q4)*sin(q5)) + dq3*(d5*cos(q2 + q3 + q4)*cos(q5) - d4*sin(q2 + q3 + q4)*sin(q5) + dc4*sin(q2 + q3 + q4)*sin(q5)) + dq4*(d5*cos(q2 + q3 + q4)*cos(q5) - d4*sin(q2 + q3 + q4)*sin(q5) + dc4*sin(q2 + q3 + q4)*sin(q5));
dJP(3,6) = (d5 - dc5)*(dq2*cos(q2 + q3 + q4)*cos(q5) + dq3*cos(q2 + q3 + q4)*cos(q5) + dq4*cos(q2 + q3 + q4)*cos(q5) - dq5*sin(q2 + q3 + q4)*sin(q5));

== matlab function control_pos_6dof_sinMI/xyz to q (referencia)/ddr to ddq ==
  data: JP input; ddq output; dJP input; dq input; ddr input
function ddq = fcn(JP,dJP,dq,ddr)

% Pseudoinversa derecha JPinv = zeros(6,3)
JPinv = JP.'*(JP*JP.')^-1;

% Aceleraciones articulares
ddq = JPinv*(ddr - dJP*dq);

== matlab function control_pos_6dof_sinMI/Inicializar posición de robot manipulador/dq_init/q4/Polinomio 7mo orden dq ==
  data: t input; q0 input; qpol output; vpol output; apol output; jpol output; q1 input; t0 input; t1 input
function [qpol,vpol,apol,jpol] = fcn(t,q0,q1,t0,t1)


% t,q0,q1,v0,v1,ac0,ac1,j0,j1,t0,t1)
%Trayectoria de referencia

% q0 = 0;
% q1 = 0;

v0 = 0;
v1 = 0;

ac0 = 0;
ac1 = 0;

j0 = 0;
j1 = 0;

% t0 = 0;
% t1 = pi/4;

% Coeficientes de un polinomio de 7mo grado

h = q1 - q0;
T = t1 - t0;

a = zeros(7+1,1);

a(1) = q0;
a(2) = v0;
a(3) = ac0/2;
a(4) = j0/6;
a(5) = (210*h-T*((30*ac0-15*ac1)*T+(4*j0+j1)*T^2+120*v0+90*v1))/(6*T^4);
a(6) = (-168*h-T*((20*ac0-14*ac1)*T+(2*j0+j1)*T^2+90*v0+78*v1))/(2*T^5);
a(7) = (420*h-T*((45*ac0-39*ac1)*T+(4*j0+3*j1)*T^2+216*v0+204*v1))/(6*T^6);
a(8) = (-120*h-T*((12*ac0-12*ac1)*T+(j0+j1)*T^2+60*v0+60*v1))/(6*T^7);

qa = flip(a')';
va = polyder(qa')';
aa = polyder(va')';
ja = polyder(aa')';


if t>=t0 && t<t1
    qpol = polyval(qa,t-t0);
    vpol = polyval(va,t-t0);
    apol = polyval(aa,t-t0);
    jpol = polyval(ja,t-t0);
elseif t>=t1
    qpol = polyval(qa,T);
    vpol = polyval(va,T);
    apol = polyval(aa,T);
    jpol = polyval(ja,T);
else
    qpol = q0;
    vpol = v0;
    apol = ac0;
    jpol = j0;
end

== matlab function control_pos_6dof_sinMI/Inicializar posición de robot manipulador/dq_init/q5/Polinomio 7mo orden dq ==
  data: t input; q0 input; qpol output; vpol output; apol output; jpol output; q1 input; t0 input; t1 input
function [qpol,vpol,apol,jpol] = fcn(t,q0,q1,t0,t1)


% t,q0,q1,v0,v1,ac0,ac1,j0,j1,t0,t1)
%Trayectoria de referencia

% q0 = 0;
% q1 = 0;

v0 = 0;
v1 = 0;

ac0 = 0;
ac1 = 0;

j0 = 0;
j1 = 0;

% t0 = 0;
% t1 = pi/4;

% Coeficientes de un polinomio de 7mo grado

h = q1 - q0;
T = t1 - t0;

a = zeros(7+1,1);

a(1) = q0;
a(2) = v0;
a(3) = ac0/2;
a(4) = j0/6;
a(5) = (210*h-T*((30*ac0-15*ac1)*T+(4*j0+j1)*T^2+120*v0+90*v1))/(6*T^4);
a(6) = (-168*h-T*((20*ac0-14*ac1)*T+(2*j0+j1)*T^2+90*v0+78*v1))/(2*T^5);
a(7) = (420*h-T*((45*ac0-39*ac1)*T+(4*j0+3*j1)*T^2+216*v0+204*v1))/(6*T^6);
a(8) = (-120*h-T*((12*ac0-12*ac1)*T+(j0+j1)*T^2+60*v0+60*v1))/(6*T^7);

qa = flip(a')';
va = polyder(qa')';
aa = polyder(va')';
ja = polyder(aa')';


if t>=t0 && t<t1
    qpol = polyval(qa,t-t0);
    vpol = polyval(va,t-t0);
    apol = polyval(aa,t-t0);
    jpol = polyval(ja,t-t0);
elseif t>=t1
    qpol = polyval(qa,T);
    vpol = polyval(va,T);
    apol = polyval(aa,T);
    jpol = polyval(ja,T);
else
    qpol = q0;
    vpol = v0;
    apol = ac0;
    jpol = j0;
end

== matlab function control_pos_6dof_sinMI/Inicializar posición de robot manipulador/dq_init1/q1/Polinomio 7mo orden dq ==
  data: t input; q0 input; qpol output; vpol output; apol output; jpol output; q1 input; t0 input; t1 input
function [qpol,vpol,apol,jpol] = fcn(t,q0,q1,t0,t1)


% t,q0,q1,v0,v1,ac0,ac1,j0,j1,t0,t1)
%Trayectoria de referencia

% q0 = 0;
% q1 = 0;

v0 = 0;
v1 = 0;

ac0 = 0;
ac1 = 0;

j0 = 0;
j1 = 0;

% t0 = 0;
% t1 = pi/4;

% Coeficientes de un polinomio de 7mo grado

h = q1 - q0;
T = t1 - t0;

a = zeros(7+1,1);

a(1) = q0;
a(2) = v0;
a(3) = ac0/2;
a(4) = j0/6;
a(5) = (210*h-T*((30*ac0-15*ac1)*T+(4*j0+j1)*T^2+120*v0+90*v1))/(6*T^4);
a(6) = (-168*h-T*((20*ac0-14*ac1)*T+(2*j0+j1)*T^2+90*v0+78*v1))/(2*T^5);
a(7) = (420*h-T*((45*ac0-39*ac1)*T+(4*j0+3*j1)*T^2+216*v0+204*v1))/(6*T^6);
a(8) = (-120*h-T*((12*ac0-12*ac1)*T+(j0+j1)*T^2+60*v0+60*v1))/(6*T^7);

qa = flip(a')';
va = polyder(qa')';
aa = polyder(va')';
ja = polyder(aa')';


if t>=t0 && t<t1
    qpol = polyval(qa,t-t0);
    vpol = polyval(va,t-t0);
    apol = polyval(aa,t-t0);
    jpol = polyval(ja,t-t0);
elseif t>=t1
    qpol = polyval(qa,T);
    vpol = polyval(va,T);
    apol = polyval(aa,T);
    jpol = polyval(ja,T);
else
    qpol = q0;
    vpol = v0;
    apol = ac0;
    jpol = j0;
end

== matlab function control_pos_6dof_sinMI/Inicializar posición de robot manipulador/dq_init1/q2/Polinomio 7mo orden dq ==
  data: t input; q0 input; qpol output; vpol output; apol output; jpol output; q1 input; t0 input; t1 input
function [qpol,vpol,apol,jpol] = fcn(t,q0,q1,t0,t1)


% t,q0,q1,v0,v1,ac0,ac1,j0,j1,t0,t1)
%Trayectoria de referencia

% q0 = 0;
% q1 = 0;

v0 = 0;
v1 = 0;

ac0 = 0;
ac1 = 0;

j0 = 0;
j1 = 0;

% t0 = 0;
% t1 = pi/4;

% Coeficientes de un polinomio de 7mo grado

h = q1 - q0;
T = t1 - t0;

a = zeros(7+1,1);

a(1) = q0;
a(2) = v0;
a(3) = ac0/2;
a(4) = j0/6;
a(5) = (210*h-T*((30*ac0-15*ac1)*T+(4*j0+j1)*T^2+120*v0+90*v1))/(6*T^4);
a(6) = (-168*h-T*((20*ac0-14*ac1)*T+(2*j0+j1)*T^2+90*v0+78*v1))/(2*T^5);
a(7) = (420*h-T*((45*ac0-39*ac1)*T+(4*j0+3*j1)*T^2+216*v0+204*v1))/(6*T^6);
a(8) = (-120*h-T*((12*ac0-12*ac1)*T+(j0+j1)*T^2+60*v0+60*v1))/(6*T^7);

qa = flip(a')';
va = polyder(qa')';
aa = polyder(va')';
ja = polyder(aa')';


if t>=t0 && t<t1
    qpol = polyval(qa,t-t0);
    vpol = polyval(va,t-t0);
    apol = polyval(aa,t-t0);
    jpol = polyval(ja,t-t0);
elseif t>=t1
    qpol = polyval(qa,T);
    vpol = polyval(va,T);
    apol = polyval(aa,T);
    jpol = polyval(ja,T);
else
    qpol = q0;
    vpol = v0;
    apol = ac0;
    jpol = j0;
end

== matlab function control_pos_6dof_sinMI/Inicializar posición de robot manipulador/dq_init1/q3/Polinomio 7mo orden dq ==
  data: t input; q0 input; qpol output; vpol output; apol output; jpol output; q1 input; t0 input; t1 input
function [qpol,vpol,apol,jpol] = fcn(t,q0,q1,t0,t1)


% t,q0,q1,v0,v1,ac0,ac1,j0,j1,t0,t1)
%Trayectoria de referencia

% q0 = 0;
% q1 = 0;

v0 = 0;
v1 = 0;

ac0 = 0;
ac1 = 0;

j0 = 0;
j1 = 0;

% t0 = 0;
% t1 = pi/4;

% Coeficientes de un polinomio de 7mo grado

h = q1 - q0;
T = t1 - t0;

a = zeros(7+1,1);

a(1) = q0;
a(2) = v0;
a(3) = ac0/2;
a(4) = j0/6;
a(5) = (210*h-T*((30*ac0-15*ac1)*T+(4*j0+j1)*T^2+120*v0+90*v1))/(6*T^4);
a(6) = (-168*h-T*((20*ac0-14*ac1)*T+(2*j0+j1)*T^2+90*v0+78*v1))/(2*T^5);
a(7) = (420*h-T*((45*ac0-39*ac1)*T+(4*j0+3*j1)*T^2+216*v0+204*v1))/(6*T^6);
a(8) = (-120*h-T*((12*ac0-12*ac1)*T+(j0+j1)*T^2+60*v0+60*v1))/(6*T^7);

qa = flip(a')';
va = polyder(qa')';
aa = polyder(va')';
ja = polyder(aa')';


if t>=t0 && t<t1
    qpol = polyval(qa,t-t0);
    vpol = polyval(va,t-t0);
    apol = polyval(aa,t-t0);
    jpol = polyval(ja,t-t0);
elseif t>=t1
    qpol = polyval(qa,T);
    vpol = polyval(va,T);
    apol = polyval(aa,T);
    jpol = polyval(ja,T);
else
    qpol = q0;
    vpol = v0;
    apol = ac0;
    jpol = j0;
end
